simulink model "FFT1"  (Simulink 7.9)
settings: Solver=ode45  StartTime=0.0  StopTime=Tsim  RelTol=1e-3
values from neighbouring files (symbols this model uses):
  Fsin = (25)*2*pi    (= 157.079632679)    [fft_script.m]    (also in script.m)
  Te = 1/Fe    (= 3.125e-06)    [Bode_partie1.m]    (also in fft_script.m = 0.03125; script.m = 0.03125; script1.m; script2.m)
settings Model: Creator=anakstel  LastModifiedBy=anakstel

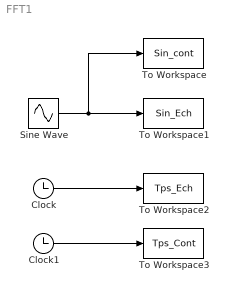
== system FFT1 ==
  Clock : Clock
  Clock1 : Clock
  Sine Wave : Sin  Frequency=Fsin  SampleTime=0
  To Workspace : ToWorkspace  VariableName=Sin_cont  SampleTime=Te/100
  To Workspace1 : ToWorkspace  VariableName=Sin_Ech  SampleTime=Te
  To Workspace2 : ToWorkspace  VariableName=Tps_Ech  SampleTime=Te
  To Workspace3 : ToWorkspace  VariableName=Tps_Cont  SampleTime=Te/100
  wires:
  Clock1/1 -> To Workspace3/1
  Clock/1 -> To Workspace2/1
  Sine Wave/1 -> To Workspace1/1, To Workspace/1
